simulink model "modified_motor"  (R2017a)
settings: Solver=FixedStepAuto  StartTime=0.0  StopTime=inf  FixedStep=0.001  RelTol=1e-3  EnableMultiTasking=on
PreLoadFcn:
  | WEBCAM_NAME = 'HP USB Webcam';
  | camera = webcam(WEBCAM_NAME);
  | 
  | load('motor_params.mat');
  | load('ui_params.mat');
  | 
  | image_data = zeros(100,3);
values from neighbouring files (symbols this model uses):
  b = 3.5077e-06    [motor_params.mat]
  J = 3.2284e-06    [motor_params.mat]
  Ke = 0.0274    [motor_params.mat]
  Kt = 0.0274    [motor_params.mat]
  L = bwlabel(binimg)    [beginning_ip.m]    (also in motor_params.mat = 0.01; test_ip2.m)
  R = 4    [motor_params.mat]
libraries: slrtlib x4, xpcquanserlib x2, simulink_extras x1
CloseFcn:
  | clear camera
settings Model: SimulationMode=external  Creator=Venkatraman  LastModifiedBy=tbirdso
settings SolverCC: EnableConcurrentExecution=on
settings DataIOCC: LimitDataPoints=on  SaveFormat=Array  LoggingToFile=on
settings OptimizationCC: BlockReduction=off  OptimizeBlockIOStorage=off  BufferReuse=off  GlobalBufferReuse=off  ExpressionFolding=off  LocalBlockOutputs=off  LifeSpan=inf
settings DebuggingCC: SolverPrmCheckMsg=warning  SFUnexpectedBacktrackingDiag=warning  SFNoUnconditionalDefaultTransitionDiag=warning  SFExecutionAtInitializationDiag=none
settings HardwareCC: ProdBitPerPointer=32  ProdBitPerSizeT=32  ProdBitPerPtrDiffT=32  ProdLargestAtomicFloat=None  ProdWordSize=32  ProdLongLongMode=on  ProdHWDeviceType=Generic->32-bit x86 compatible  TargetBitPerPointer=64  TargetBitPerSizeT=64  TargetBitPerPtrDiffT=64  TargetLongLongMode=on  TargetIntDivRoundTo=Zero  TargetEndianess=LittleEndian  TargetWordSize=64  TargetHWDeviceType=MATLAB Host
settings ModelReferenceCC: PropagateSignalLabelsOutOfModel=off
settings RTWCC: SystemTargetFile=slrt.tlc  TemplateMakefile=slrt_default_tmf  Description=Simulink Real-Time  RTWVerbose=off  RTWCompilerOptimization=on
settings SimulinkRealTimeCC: GeneratePreprocessorConditionals=Disable all
settings ConfigComp: CovMetricSettings=dw  CovHtmlReporting=on  CovSaveCumulativeToWorkspaceVar=on  CovSaveSingleToWorkspaceVar=on  CovExternalEMLEnable=off  CovSFcnEnable=off

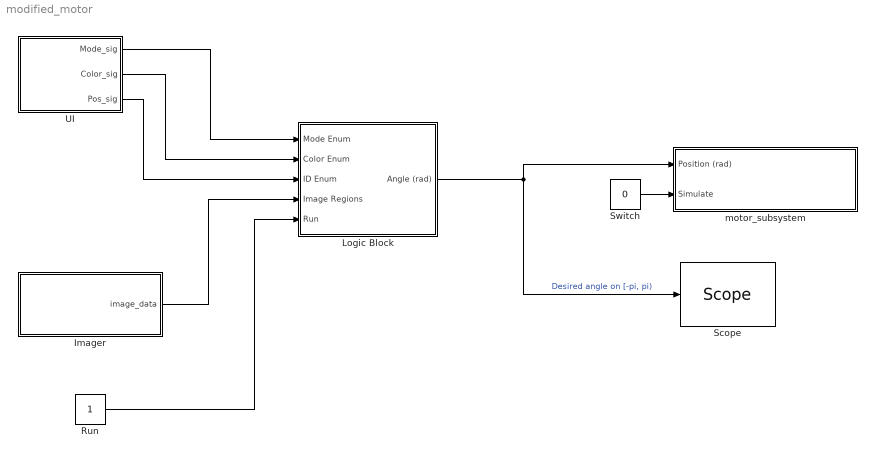
== system modified_motor ==
  Imager : Subsystem
  Logic Block : Subsystem
  Run : Constant
  "Scope " : slrtlib/Displays and Logging/Scope   scopeno=3  scopetype=Target  autostart=on  viewmode=Numerical  formatstr='%15.6f'  grid=on  ylimits=[0,0]  nosamples=250  noprepostsamples=0  interleave=1  triggermode=Scope triggering  triggersignal=1  trigsignalfromport=off  triggerlevel=0.0  triggerslope=Either  triggerscope=1  triggersample=0  filename=data.dat  mode=Lazy  writesize=512  autorestart=off  dynamicfilemode=off  maxwritefilesize=512*1024^2
  Switch : Constant  Value=0
  UI : Subsystem
  motor_subsystem : Subsystem
  wires:
  Logic Block/1(Angle (rad)) -> "Scope "/1, motor_subsystem/1(Position (rad))  "Desired angle on [-pi, pi)"
  UI/1(Mode_sig) -> Logic Block/1(Mode Enum)
  UI/2(Color_sig) -> Logic Block/2(Color Enum)
  UI/3(Pos_sig) -> Logic Block/3(ID Enum)
  Imager/1(image_data) -> Logic Block/4(Image Regions)
  Switch/1 -> motor_subsystem/2(Simulate)
  Run/1 -> Logic Block/5(Run)

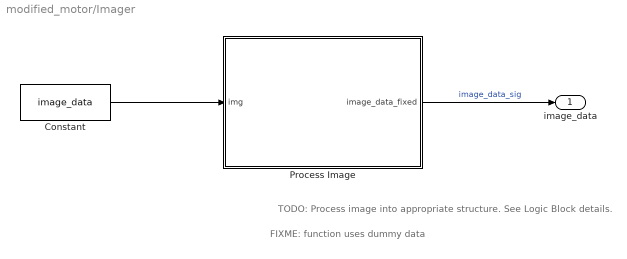
== system modified_motor/Imager ==
  note: FIXME: function uses dummy data
  note: TODO: Process image into appropriate structure. See Logic Block details.
  Constant : Constant  Value=image_data
  Process Image : MATLAB Function  TreatAsAtomicUnit=on
  image_data : Outport
  wires:
  Process Image/1(image_data_fixed) -> image_data/1  "image_data_sig"
  Constant/1 -> Process Image/1(img)

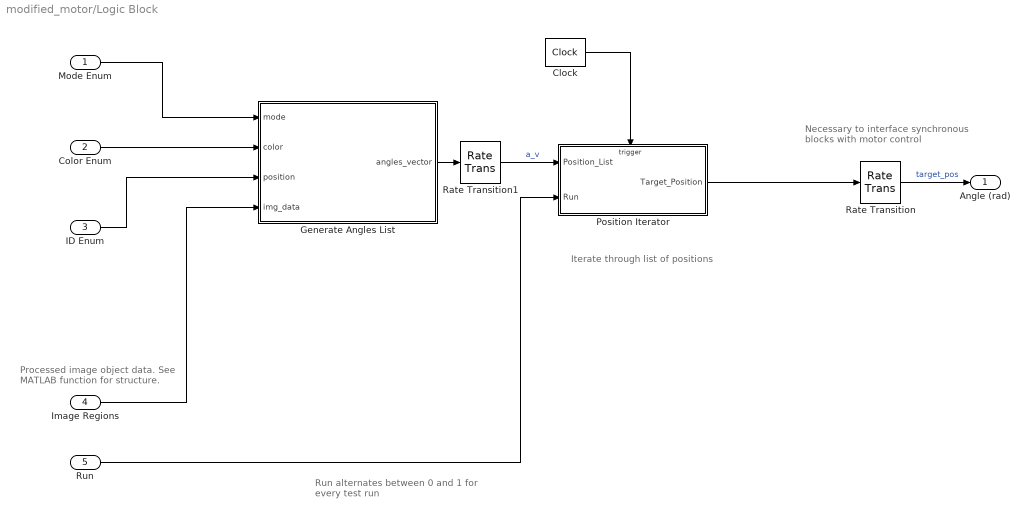
== system modified_motor/Logic Block ==
  note: Necessary to interface synchronous
      | blocks with motor control
  note: Iterate through list of positions
  note: Processed image object data.
      | See MATLAB function for structure.
  note: Run alternates between 0 and 1 for every test run
  Mode Enum : Inport
  Color Enum : Inport  Port=2
  ID Enum : Inport  Port=3
  Image Regions : Inport  Port=4
  Run : Inport  Port=5
  Clock : simulink_extras/Flip Flops/Clock  period=2
  Generate Angles List : MATLAB Function  TreatAsAtomicUnit=on
  Position Iterator : Subsystem  TreatAsAtomicUnit=on
  Rate Transition : RateTransition
  Rate Transition1 : RateTransition
  Angle (rad) : Outport
  wires:
  Mode Enum/1 -> Generate Angles List/1(mode)
  Color Enum/1 -> Generate Angles List/2(color)
  ID Enum/1 -> Generate Angles List/3(position)
  Image Regions/1 -> Generate Angles List/4(img_data)
  Position Iterator/1(Target_Position) -> Rate Transition/1
  Clock/1 -> Position Iterator/Trigger
  Run/1 -> Position Iterator/2(Run)
  Generate Angles List/1(angles_vector) -> Rate Transition1/1
  Rate Transition/1 -> Angle (rad)/1  "target_pos"
  Rate Transition1/1 -> Position Iterator/1(Position_List)  "a_v"

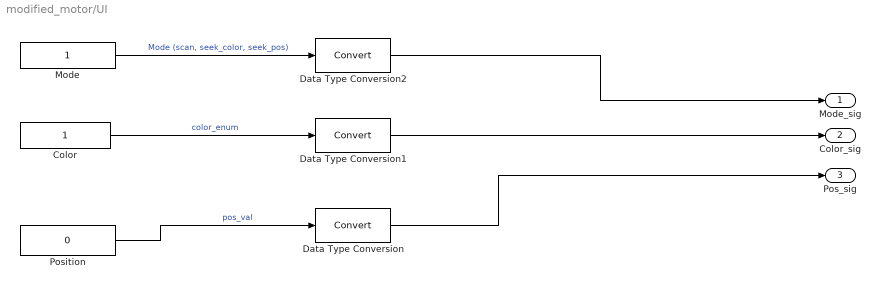
== system modified_motor/UI ==
  Color : Constant
  Data Type Conversion : DataTypeConversion
  Data Type Conversion1 : DataTypeConversion
  Data Type Conversion2 : DataTypeConversion
  Mode : Constant  OutDataTypeStr=int8
  Position : Constant  Value=0
  Mode_sig : Outport
  Color_sig : Outport  Port=2
  Pos_sig : Outport  Port=3
  wires:
  Mode/1 -> Data Type Conversion2/1  "Mode (scan, seek_color, seek_pos)"
  Color/1 -> Data Type Conversion1/1  "color_enum"
  Data Type Conversion/1 -> Pos_sig/1
  Position/1 -> Data Type Conversion/1  "pos_val"
  Data Type Conversion1/1 -> Color_sig/1
  Data Type Conversion2/1 -> Mode_sig/1

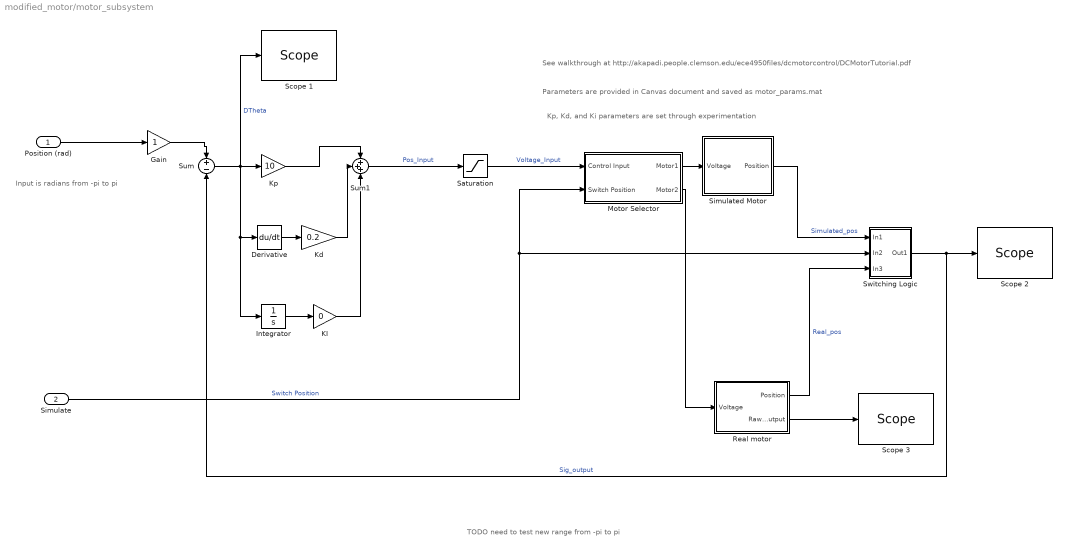
== system modified_motor/motor_subsystem ==
  note: TODO need to test new range from -pi to pi
  note: Kp, Kd, and Ki parameters are set through experimentation
  note: Parameters are provided in Canvas document and saved as motor_params.mat
  note: See walkthrough at http://akapadi.people.clemson.edu/ece4950files/dcmotorcontrol/DCMotorTutorial.pdf
  note: Input is radians from -pi to pi
  Position (rad) : Inport
  Simulate : Inport  Port=2
  Derivative : Derivative
  Gain : Gain
  Integrator : Integrator
  KI : Gain  Gain=0
  Kd : Gain  Gain=0.2
  Kp : Gain  Gain=10
  Motor Selector : Subsystem
  Real motor : Subsystem
  Saturation : Saturate  UpperLimit=5  LowerLimit=-5
  Scope 1 : slrtlib/Displays and Logging/Scope   scopeno=2  scopetype=Target  autostart=on  viewmode=Graphical redraw  formatstr='%15.6f'  grid=on  ylimits=[0,2]  nosamples=250  noprepostsamples=0  interleave=1  triggermode=FreeRun  triggersignal=1  trigsignalfromport=off  triggerlevel=0.0  triggerslope=Either  triggerscope=1  triggersample=0  filename=data.dat  mode=Lazy  writesize=512  autorestart=off  dynamicfilemode=off  maxwritefilesize=512*1024^2
  Scope 2 : slrtlib/Displays and Logging/Scope   scopeno=1  scopetype=Target  autostart=on  viewmode=Numerical  formatstr='%15.6f'  grid=on  ylimits=[0,2]  nosamples=250  noprepostsamples=0  interleave=1  triggermode=FreeRun  triggersignal=1  trigsignalfromport=off  triggerlevel=0.0  triggerslope=Either  triggerscope=1  triggersample=0  filename=data.dat  mode=Lazy  writesize=512  autorestart=off  dynamicfilemode=off  maxwritefilesize=512*1024^2
  Scope 3 : slrtlib/Displays and Logging/Scope   scopeno=4  scopetype=Target  autostart=on  viewmode=Numerical  formatstr='%15.6f'  grid=on  ylimits=[0,2]  nosamples=250  noprepostsamples=0  interleave=1  triggermode=FreeRun  triggersignal=1  trigsignalfromport=off  triggerlevel=0.0  triggerslope=Either  triggerscope=1  triggersample=0  filename=data.dat  mode=Lazy  writesize=512  autorestart=off  dynamicfilemode=off  maxwritefilesize=512*1024^2
  Simulated Motor : Subsystem
  Sum : Sum  Inputs=+-
  Sum1 : Sum  Inputs=+++
  Switching Logic : Subsystem
  wires:
  Real motor/1(Position) -> Switching Logic/3(In3)  "Real_pos"
  Sum1/1 -> Saturation/1  "Pos_Input"
  Derivative/1 -> Kd/1
  Integrator/1 -> KI/1
  Sum/1 -> Integrator/1, Derivative/1, Scope 1/1, Kp/1  "DTheta"
  Motor Selector/2(Motor2) -> Real motor/1(Voltage)
  KI/1 -> Sum1/3
  Switching Logic/1(Out1) -> Scope 2/1, Sum/2  "Sig_output"
  Position (rad)/1 -> Gain/1
  Real motor/2(Raw Output) -> Scope 3/1
  Motor Selector/1(Motor1) -> Simulated Motor/1(Voltage)
  Saturation/1 -> Motor Selector/1(Control Input)  "Voltage_Input"
  Kp/1 -> Sum1/1
  Gain/1 -> Sum/1
  Simulated Motor/1(Position) -> Switching Logic/1(In1)  "Simulated_pos"
  Simulate/1 -> Switching Logic/2(In2), Motor Selector/2(Switch Position)  "Switch Position"
  Kd/1 -> Sum1/2

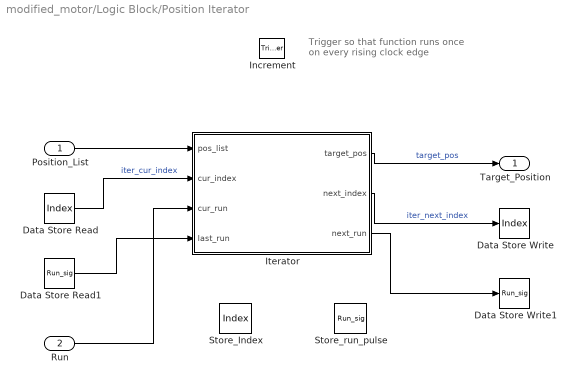
== system modified_motor/Logic Block/Position Iterator ==
  note: Trigger so that function runs
      | once on every rising clock edge
  Position_List : Inport
  Run : Inport  Port=2
  Increment : TriggerPort  VariantControl=Variant  InitialTriggerSignalState=zero
  Data Store Read : DataStoreRead  DataStoreName=Index
  Data Store Read1 : DataStoreRead  DataStoreName=Run_sig
  Data Store Write : DataStoreWrite  DataStoreName=Index
  Data Store Write1 : DataStoreWrite  DataStoreName=Run_sig
  Iterator : MATLAB Function  TreatAsAtomicUnit=on
  Store_Index : DataStoreMemory  DataStoreName=Index  ReadBeforeWriteMsg=warning  WriteAfterWriteMsg=warning  WriteAfterReadMsg=warning  InitialValue=99  ShowAdditionalParam=off
  Store_run_pulse : DataStoreMemory  DataStoreName=Run_sig  ReadBeforeWriteMsg=warning  WriteAfterWriteMsg=warning  WriteAfterReadMsg=warning  ShowAdditionalParam=off
  Target_Position : Outport
  wires:
  Position_List/1 -> Iterator/1(pos_list)
  Iterator/1(target_pos) -> Target_Position/1  "target_pos"
  Run/1 -> Iterator/3(cur_run)
  Data Store Read/1 -> Iterator/2(cur_index)  "iter_cur_index"
  Iterator/2(next_index) -> Data Store Write/1  "iter_next_index"
  Data Store Read1/1 -> Iterator/4(last_run)
  Iterator/3(next_run) -> Data Store Write1/1

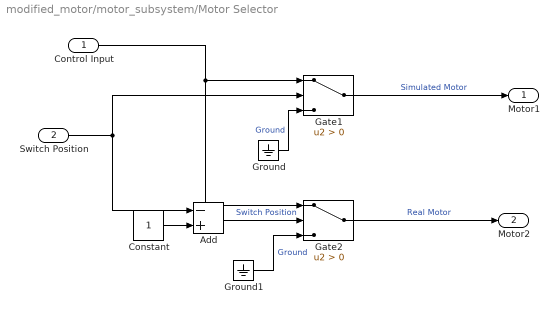
== system modified_motor/motor_subsystem/Motor Selector ==
  Control Input : Inport
  Switch Position : Inport  Port=2
  Add : Sum  Inputs=-+
  Constant : Constant
  Gate1 : Switch  Criteria=u2 > Threshold
  Gate2 : Switch  Criteria=u2 > Threshold
  Ground : Ground
  Ground1 : Ground
  Motor1 : Outport
  Motor2 : Outport  Port=2
  wires:
  Gate1/1 -> Motor1/1  "Simulated Motor"
  Ground/1 -> Gate1/3  "Ground"
  Control Input/1 -> Gate2/1, Gate1/1
  Add/1 -> Gate2/2  "Switch Position"
  Ground1/1 -> Gate2/3  "Ground"
  Gate2/1 -> Motor2/1  "Real Motor"
  Switch Position/1 -> Add/1, Gate1/2
  Constant/1 -> Add/2

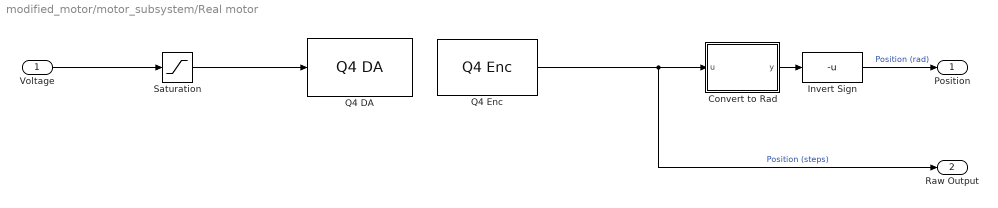
== system modified_motor/motor_subsystem/Real motor ==
  Voltage : Inport
  Convert to Rad : MATLAB Function  TreatAsAtomicUnit=on
  Invert Sign : Fcn  Expr=-u
  "Q4 DA " : xpcquanserlib/D//A/Q4 DA   channel=[1]  range=[-5]  simul=off  reset=[1]  initValue=[0]  sampleTime=.001  slot=-1
      settings: SourceProductName=Simulink Real-Time  SourceProductBaseCode=XP
  "Q4 Enc " : xpcquanserlib/Incremental Encoder/Q4 Enc   channel=[1]  initialCount=[0]  prescale=[1]  quadrature=[1]  mode=[0]  synchronousIndex=[0]  indexPolarity=[0]  preserveCounts=[0]  sampleTime=.001  slot=-1
      settings: SourceProductName=Simulink Real-Time  SourceProductBaseCode=XP
  Saturation : Saturate  UpperLimit=5  LowerLimit=-5
  Position : Outport
  Raw Output : Outport  Port=2
  wires:
  Voltage/1 -> Saturation/1
  "Q4 Enc "/1 -> Raw Output/1, Convert to Rad/1(u)  "Position (steps)"
  Saturation/1 -> "Q4 DA "/1
  Invert Sign/1 -> Position/1  "Position (rad)"
  Convert to Rad/1(y) -> Invert Sign/1

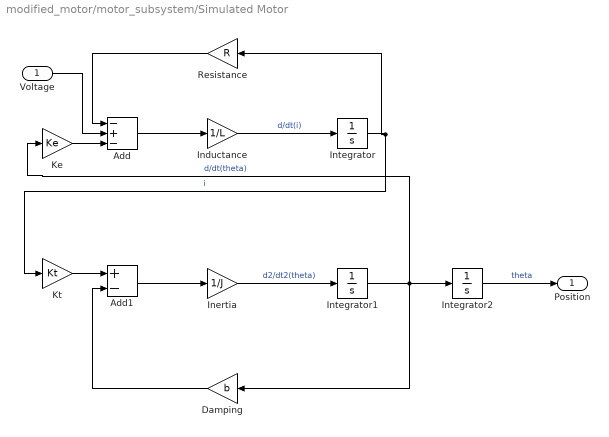
== system modified_motor/motor_subsystem/Simulated Motor ==
  Voltage : Inport
  Add : Sum  Inputs=-+-
  Add1 : Sum  Inputs=+-
  Damping : Gain  Gain=b
  Inductance : Gain  Gain=1/L
  "Inertia " : Gain  Gain=1/J
  Integrator : Integrator
  Integrator1 : Integrator
  Integrator2 : Integrator
  Ke : Gain  Gain=Ke
  Kt : Gain  Gain=Kt
  Resistance : Gain  Gain=R
  Position : Outport
  wires:
  Resistance/1 -> Add/1
  Ke/1 -> Add/3
  Kt/1 -> Add1/1
  Integrator/1 -> Resistance/1, Kt/1  "i"
  Add/1 -> Inductance/1
  Voltage/1 -> Add/2
  Integrator2/1 -> Position/1  "theta"
  Integrator1/1 -> Ke/1, Damping/1, Integrator2/1  "d/dt(theta)"
  Inductance/1 -> Integrator/1  "d/dt(i)"
  "Inertia "/1 -> Integrator1/1  "d2/dt2(theta)"
  Damping/1 -> Add1/2
  Add1/1 -> "Inertia "/1

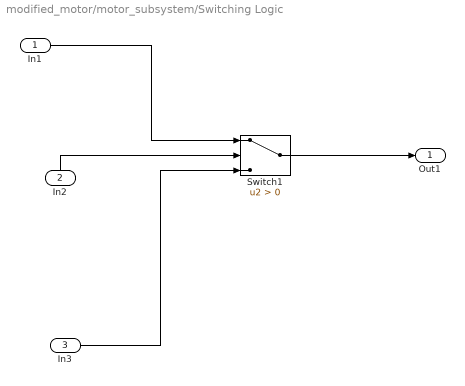
== system modified_motor/motor_subsystem/Switching Logic ==
  In1 : Inport
  In2 : Inport  Port=2
  In3 : Inport  Port=3
  Switch1 : Switch  Criteria=u2 > Threshold
  Out1 : Outport
  wires:
  In3/1 -> Switch1/3
  Switch1/1 -> Out1/1
  In1/1 -> Switch1/1
  In2/1 -> Switch1/2

== matlab function modified_motor/Logic Block/Generate Angles List ==
  data: mode input; angles_vector output; color input; position input; img_data input
% PURPOSE - Parser to set 
% INPUTS
%   - Mode: What should the system do in response to the user selection
%       - scan: Visit every well with a sticker
%       - seek color: Visit every well with a sticker of the given color
%       - seek position: Visit only the well with the given sticker ID
%   - Color Enum: What color the system should visit
%   - Position: Angle in radians to visit
%   - Image Data: 2D processed data from webcam
%       - Col 1: Color
%       - Col 2: X Position
%       - Col 3: Y Position
% OUTPUTS
%   - positions_to_visit: Vector of fixed destination positions on [-pi, pi) 
%       to which the motor arm should point in sequence.
% NOTES
%   - If mode = 1 then the function ignores requested position and color.
%   - If mode = 2 then the function ignores requested position.
%   - If mode = 3 then the function ignores requested color.


function angles_vector = make_angle_vector(mode, color, position, img_data)

% MATLAB expects a fixed-size output matrix so allow up to 100 angles
% to be propagated
MAX_ANGLES_TO_VISIT = 100;

MODE_SCAN = 1;
MODE_SEEK_COLOR = 2;
MODE_SEEK_POSITION = 3;

COLOR_COL = 1;
X_COL = 2;
Y_COL = 3;

angles_vector = zeros(MAX_ANGLES_TO_VISIT, 1);

if mode == MODE_SCAN
    rect_coords = img_data(img_data(:,1) ~= 0, X_COL:Y_COL);
    angles_to_visit = rect_to_polar_v2(rect_coords);

elseif mode == MODE_SEEK_COLOR
    rect_coords = img_data(img_data(:, COLOR_COL) == color, X_COL:Y_COL);
    angles_to_visit = rect_to_polar_v2(rect_coords);

elseif mode == MODE_SEEK_POSITION
    angles_to_visit = position;

else
    angles_to_visit = [pi; -pi; pi/2; -pi/2];
end

% Package variable-length vector into fixed-length vector
angles_vector(1:size(angles_to_visit,1), :) = angles_to_visit;

== matlab function modified_motor/motor_subsystem/Real motor/Convert to Rad ==
  data: u input; y output
function y = fcn(u)

% Observed experimentally
STEPS_IN_ONE_ROTATION = 400;

rads_from_zero_to_twopi = u * 2 * pi / STEPS_IN_ONE_ROTATION;

y = rads_from_zero_to_twopi;

== matlab function modified_motor/Imager/Process Image ==
  data: image_data_fixed output; img input
function image_data_fixed = process_image(img)

% Can only send fixed-length matrices so specify max 100 regions
REGIONS_SIGNAL_CAPACITY = 100;

% FIXME do processing
image_data_fixed = zeros(REGIONS_SIGNAL_CAPACITY, 3);

% ex. pass back [shape; color; x_pos; y_pos]
image_data_fixed(1:size(img,1),:) = img;

== matlab function modified_motor/Logic Block/Position Iterator/Iterator ==
  data: pos_list input; cur_index input; target_pos output; next_index output; cur_run input; last_run input; next_run output
% PURPOSE - Iterate over list of positions to visit
% INPUTS
%   - Position List: Vector of target positions for the motor to turn to
%   - Current Index: Loopback to store variable state
%   - Clock: Trigger to move to the next position
%   - Reset: Trigger to reset to first position in list (0 == HIGH)
% OUTPUTS
%   - Target Position: Motor position on range [-pi, pi) 
%   - Next Index: Loopback to store variable state
% BEHAVIOR
%   - If Reset is high then reset index to 0 and output first position
%   - Else if Clock is low then output the position at the current index
%   - Else if the index is at the end of the list then output 0
%   - Else increment the index and output the next position

function [target_pos, next_index, next_run] = iterate(pos_list, cur_index, cur_run, last_run)

% PRECONDITION: pos_list is a column vector
assert(size(pos_list, 2) == 1)

ZERO_POSITION = 0;
pos_list_len = size(pos_list, 1);

% This is a very hack-y edge trigger
if cur_run ~= last_run
   next_index = 1;
   target_pos = pos_list(1);
else
   % If we can increment then do that
    if -1 < cur_index && cur_index < pos_list_len
        next_index = cur_index + 1;
        target_pos = pos_list(cur_index + 1);
    % Otherwise maintain current state
    else
        next_index = cur_index;
        target_pos = ZERO_POSITION;
    end
end

next_run = cur_run;
